simulink model "Halfcar_model_EV_simulink"  (Simulink 7.3)
settings: Solver=ode3  StartTime=0.0  StopTime=5  FixedStep=T  RelTol=1e-3
values from neighbouring files (symbols this model uses):
  v_initial = 10    [Main_for_DOCandDODR.m]
undefined symbols (not defined in the file or in its folder): a, b, cf, cr, Ds, eyeb, eyew, g, h, kf, kr, ktf, ktr, M1, M2, mb, mw, r, reduction_ratio, saturation_slipratio, step_time, T, Tdf, Tdr, wf_initial, wr_initial
libraries: simulink x2
settings Model: Creator=JSP  LastModifiedBy=JSPark

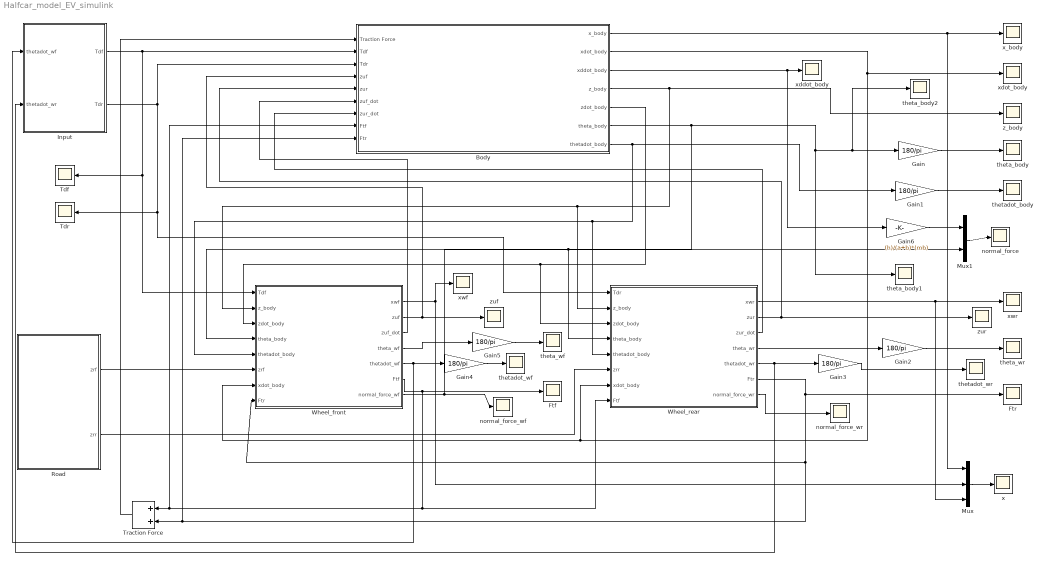
== system Halfcar_model_EV_simulink ==
  Body : Subsystem
  Ftf : Scope
      settings: YMin=1706.26  YMax=1706.26  SaveName=ScopeData11
  Ftr : Scope
      settings: SaveName=ScopeData12
  Gain{,1..5} (6 alike) : Gain  Gain=180/pi  ParameterDataType=fixdt(1, 16)  ParameterScaling=2^0  OutDataType=fixdt(1, 16)  OutScaling=2^0  SampleTime=T
  Gain6 : Gain  Gain=(h)/(a+b)*(mb)  ParameterDataType=fixdt(1, 16)  ParameterScaling=2^0  OutDataType=fixdt(1, 16)  OutScaling=2^0  SampleTime=T
  Input : Subsystem
  Mux : Mux  Inputs=3
  Mux1 : Mux  Inputs=2
  Road : Subsystem
  Tdf : Scope
      settings: YMin=-315  YMax=-285  SaveName=ScopeData24
  Tdr : Scope
      settings: SaveName=ScopeData25
  Traction Force : Sum  OutDataType=fixdt(1, 16)  OutScaling=2^-10  SampleTime=T
  Wheel_front : Subsystem
  Wheel_rear : Subsystem
  normal_force : Scope
      settings: SaveName=ScopeData33
  normal_force_wf : Scope
      settings: YMin=0  YMax=400  SaveName=ScopeData26
  normal_force_wr : Scope
      settings: SaveName=ScopeData27
  theta_body : Scope
      settings: YMin=-0.5  YMax=0  SaveName=ScopeData3
  theta_body1 : Scope
      settings: YMin=-0.5  YMax=0  SaveName=ScopeData32
  theta_body2 : Scope
      settings: YMin=-0.5  YMax=0  SaveName=ScopeData34
  theta_wf : Scope
      settings: SaveName=ScopeData8
  theta_wr : Scope
      settings: SaveName=ScopeData6
  thetadot_body : Scope
      settings: SaveName=ScopeData4
  thetadot_wf : Scope
      settings: SaveName=ScopeData18
  thetadot_wr : Scope
      settings: SaveName=ScopeData17
  x : Scope
      settings: SaveName=ScopeData13
  x_body : Scope
      settings: YMin=0  YMax=250
  xddot_body : Scope
      settings: YMin=10.125  YMax=10.45  SaveName=ScopeData28
  xdot_body : Scope
      settings: YMin=10  YMax=22
  xwf : Scope
      settings: SaveName=ScopeData9
  xwr : Scope
      settings: SaveName=ScopeData5
  z_body : Scope
      settings: YMin=0.00525  YMax=0.0075  SaveName=ScopeData2
  zuf : Scope
      settings: YMin=-1  YMax=1  SaveName=ScopeData10
  zur : Scope
      settings: SaveName=ScopeData7
  wires:
  Input/1(Tdf) -> Body/2(Tdf), Tdf/1, Wheel_front/1(Tdf)
  Input/2(Tdr) -> Body/3(Tdr), Wheel_rear/1(Tdr), Tdr/1
  Road/1(zrf) -> Wheel_front/6(zrf)
  Road/2(zrr) -> Wheel_rear/6(zrr)
  Body/4(z_body) -> Wheel_front/2(z_body), Wheel_rear/2(z_body), z_body/1
  Body/6(theta_body) -> Wheel_front/4(theta_body), Wheel_rear/4(theta_body), theta_body1/1, Gain/1, theta_body2/1
  Wheel_front/2(zuf) -> Body/4(zuf), zuf/1
  Wheel_rear/2(zur) -> Body/5(zur), zur/1
  Body/1(x_body) -> x_body/1, Mux/1
  Body/2(xdot_body) -> xdot_body/1, Wheel_front/7(xdot_body), Wheel_rear/7(xdot_body)
  Body/7(thetadot_body) -> Gain1/1, Wheel_front/5(thetadot_body), Wheel_rear/5(thetadot_body)
  Wheel_rear/1(xwr) -> xwr/1, Mux/3
  Wheel_rear/4(theta_wr) -> Gain2/1
  Wheel_front/1(xwf) -> xwf/1, Mux/2
  Wheel_front/4(theta_wf) -> Gain5/1
  Wheel_front/6(Ftf) -> Ftf/1, Wheel_rear/8(Ftf), Traction Force/1, Body/8(Ftf)
  Traction Force/1 -> Body/1(Traction Force)
  Wheel_rear/6(Ftr) -> Ftr/1, Wheel_front/8(Ftr), Traction Force/2, Body/9(Ftr)
  Mux/1 -> x/1
  Wheel_rear/5(thetadot_wr) -> Gain3/1, Input/2(thetadot_wr)
  Wheel_front/5(thetadot_wf) -> Gain4/1, Input/1(thetadot_wf)
  Gain/1 -> theta_body/1
  Gain1/1 -> thetadot_body/1
  Gain2/1 -> theta_wr/1
  Gain3/1 -> thetadot_wr/1
  Gain4/1 -> thetadot_wf/1
  Gain5/1 -> theta_wf/1
  Wheel_front/3(zuf_dot) -> Body/6(zuf_dot)
  Wheel_rear/3(zur_dot) -> Body/7(zur_dot)
  Body/5(zdot_body) -> Wheel_front/3(zdot_body), Wheel_rear/3(zdot_body)
  Wheel_front/7(normal_force_wf) -> normal_force_wf/1, Mux1/2
  Wheel_rear/7(normal_force_wr) -> normal_force_wr/1
  Body/3(xddot_body) -> xddot_body/1, Gain6/1
  Gain6/1 -> Mux1/1
  Mux1/1 -> normal_force/1

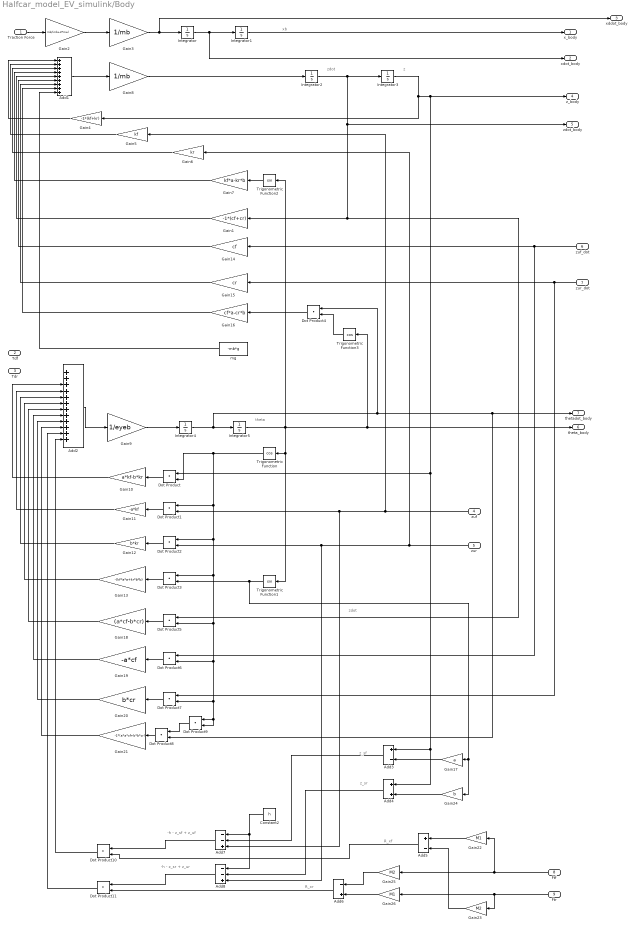
== system Halfcar_model_EV_simulink/Body ==
  note: xb
  note: z
  note: theta
  note: zdot
  note: zdot
  note: R_xf
  note: R_xr
  note: z_sf
  note: z_sr
  note: -h - z_sf + z_uf
  note: -h - z_sr + z_ur
  Traction Force : Inport
  Tdf : Inport  Port=2
  Tdr : Inport  Port=3
  zuf : Inport  Port=4
  zur : Inport  Port=5
  zuf_dot : Inport  Port=6
  zur_dot : Inport  Port=7
  Ftf : Inport  Port=8
  Ftr : Inport  Port=9
  Add1 : Sum  Inputs=+++++++++  OutDataType=fixdt(1, 16)  OutScaling=2^-10  SampleTime=T
  Add2 : Sum  Inputs=++++++++++++  OutDataType=fixdt(1, 16)  OutScaling=2^-10  SampleTime=T
  Add3 : Sum  Inputs=+-  OutDataType=fixdt(1, 16)  OutScaling=2^-10  SampleTime=T
  Add4 : Sum  OutDataType=fixdt(1, 16)  OutScaling=2^-10  SampleTime=T
  Add5 : Sum  Inputs=+-  OutDataType=fixdt(1, 16)  OutScaling=2^-10  SampleTime=T
  Add6 : Sum  Inputs=-+  OutDataType=fixdt(1, 16)  OutScaling=2^-10  SampleTime=T
  Add7 : Sum  Inputs=--+  OutDataType=fixdt(1, 16)  OutScaling=2^-10  SampleTime=T
  Add8 : Sum  Inputs=--+  OutDataType=fixdt(1, 16)  OutScaling=2^-10  SampleTime=T
  Constant2 : Constant  Value=h  OutDataType=fixdt(1, 16)  OutScaling=2^0  SampleTime=T
  Dot Product{,1..11} (12 alike) : DotProduct  SampleTime=T  OutDataType=fixdt(1, 16)  OutScaling=2^-10  InputSameDT=on  OutDataTypeStr=Inherit: Inherit via internal rule
  Gain1 : Gain  Gain=-1*(cf+cr)  ParameterDataType=fixdt(1, 16)  ParameterScaling=2^0  OutDataType=fixdt(1, 16)  OutScaling=2^0  SampleTime=T
  Gain10 : Gain  Gain=a*kf-b*kr  ParameterDataType=fixdt(1, 16)  ParameterScaling=2^0  OutDataType=fixdt(1, 16)  OutScaling=2^0  SampleTime=T
  Gain11 : Gain  Gain=-a*kf  ParameterDataType=fixdt(1, 16)  ParameterScaling=2^0  OutDataType=fixdt(1, 16)  OutScaling=2^0  SampleTime=T
  Gain12 : Gain  Gain=b*kr  ParameterDataType=fixdt(1, 16)  ParameterScaling=2^0  OutDataType=fixdt(1, 16)  OutScaling=2^0  SampleTime=T
  Gain13 : Gain  Gain=-(kf*a*a+kr*b*b)  ParameterDataType=fixdt(1, 16)  ParameterScaling=2^0  OutDataType=fixdt(1, 16)  OutScaling=2^0  SampleTime=T
  Gain14 : Gain  Gain=cf  ParameterDataType=fixdt(1, 16)  ParameterScaling=2^0  OutDataType=fixdt(1, 16)  OutScaling=2^0  SampleTime=T
  Gain15 : Gain  Gain=cr  ParameterDataType=fixdt(1, 16)  ParameterScaling=2^0  OutDataType=fixdt(1, 16)  OutScaling=2^0  SampleTime=T
  Gain16 : Gain  Gain=cf*a-cr*b  ParameterDataType=fixdt(1, 16)  ParameterScaling=2^0  OutDataType=fixdt(1, 16)  OutScaling=2^0  SampleTime=T
  Gain17 : Gain  Gain=a  ParameterDataType=fixdt(1, 16)  ParameterScaling=2^0  OutDataType=fixdt(1, 16)  OutScaling=2^0  SampleTime=T
  Gain18 : Gain  Gain=(a*cf-b*cr)  ParameterDataType=fixdt(1, 16)  ParameterScaling=2^0  OutDataType=fixdt(1, 16)  OutScaling=2^0  SampleTime=T
  Gain19 : Gain  Gain=-a*cf  ParameterDataType=fixdt(1, 16)  ParameterScaling=2^0  OutDataType=fixdt(1, 16)  OutScaling=2^0  SampleTime=T
  Gain2 : Gain  Gain=mb/(mb+2*mw)  ParameterDataType=fixdt(1, 16)  ParameterScaling=2^0  OutDataType=fixdt(1, 16)  OutScaling=2^0  SampleTime=T
  Gain20 : Gain  Gain=b*cr  ParameterDataType=fixdt(1, 16)  ParameterScaling=2^0  OutDataType=fixdt(1, 16)  OutScaling=2^0  SampleTime=T
  Gain21 : Gain  Gain=-1*(a*a*cf+b*b*cr)  ParameterDataType=fixdt(1, 16)  ParameterScaling=2^0  OutDataType=fixdt(1, 16)  OutScaling=2^0  SampleTime=T
  Gain22 : Gain  Gain=M1  ParameterDataType=fixdt(1, 16)  ParameterScaling=2^0  OutDataType=fixdt(1, 16)  OutScaling=2^0  SampleTime=T
  Gain23 : Gain  Gain=M2  ParameterDataType=fixdt(1, 16)  ParameterScaling=2^0  OutDataType=fixdt(1, 16)  OutScaling=2^0  SampleTime=T
  Gain24 : Gain  Gain=b  ParameterDataType=fixdt(1, 16)  ParameterScaling=2^0  OutDataType=fixdt(1, 16)  OutScaling=2^0  SampleTime=T
  Gain25 : Gain  Gain=M2  ParameterDataType=fixdt(1, 16)  ParameterScaling=2^0  OutDataType=fixdt(1, 16)  OutScaling=2^0  SampleTime=T
  Gain26 : Gain  Gain=M1  ParameterDataType=fixdt(1, 16)  ParameterScaling=2^0  OutDataType=fixdt(1, 16)  OutScaling=2^0  SampleTime=T
  Gain3 : Gain  Gain=1/mb  ParameterDataType=fixdt(1, 16)  ParameterScaling=2^0  OutDataType=fixdt(1, 16)  OutScaling=2^0  SampleTime=T
  Gain4 : Gain  Gain=-1*(kf+kr)  ParameterDataType=fixdt(1, 16)  ParameterScaling=2^0  OutDataType=fixdt(1, 16)  OutScaling=2^0  SampleTime=T
  Gain5 : Gain  Gain=kf  ParameterDataType=fixdt(1, 16)  ParameterScaling=2^0  OutDataType=fixdt(1, 16)  OutScaling=2^0  SampleTime=T
  Gain6 : Gain  Gain=kr  ParameterDataType=fixdt(1, 16)  ParameterScaling=2^0  OutDataType=fixdt(1, 16)  OutScaling=2^0  SampleTime=T
  Gain7 : Gain  Gain=kf*a-kr*b  ParameterDataType=fixdt(1, 16)  ParameterScaling=2^0  OutDataType=fixdt(1, 16)  OutScaling=2^0  SampleTime=T
  Gain8 : Gain  Gain=1/mb  ParameterDataType=fixdt(1, 16)  ParameterScaling=2^0  OutDataType=fixdt(1, 16)  OutScaling=2^0  SampleTime=T
  Gain9 : Gain  Gain=1/eyeb  ParameterDataType=fixdt(1, 16)  ParameterScaling=2^0  OutDataType=fixdt(1, 16)  OutScaling=2^0  SampleTime=T
  Integrator : Integrator  InitialCondition=v_initial
  Integrator{1..5} (5 alike) : Integrator
  Trigonometric Function : Trigonometry  Operator=cos  SampleTime=T
  Trigonometric Function1 : Trigonometry  SampleTime=T
  Trigonometric Function2 : Trigonometry  SampleTime=T
  Trigonometric Function3 : Trigonometry  Operator=cos  SampleTime=T
  mg : Constant  Value=-mb*g  OutDataType=fixdt(1, 16)  OutScaling=2^0  SampleTime=T
  x_body : Outport
  xdot_body : Outport  Port=2
  xddot_body : Outport  Port=3
  z_body : Outport  Port=4
  zdot_body : Outport  Port=5
  theta_body : Outport  Port=6
  thetadot_body : Outport  Port=7
  wires:
  Gain2/1 -> Gain3/1
  Gain3/1 -> Integrator/1, xddot_body/1
  Integrator/1 -> Integrator1/1, xdot_body/1
  Gain8/1 -> Integrator2/1
  Integrator2/1 -> Integrator3/1, Gain1/1, Dot Product5/1, zdot_body/1
  Add1/1 -> Gain8/1
  Gain4/1 -> Add1/1
  Gain5/1 -> Add1/2
  Gain6/1 -> Add1/3
  Gain7/1 -> Add1/4
  Integrator3/1 -> Gain4/1, z_body/1, Dot Product/1, Add3/1, Add4/1
  Gain9/1 -> Integrator4/1
  Integrator4/1 -> Integrator5/1, Dot Product4/1, thetadot_body/1, Dot Product8/2
  Dot Product/1 -> Gain10/1
  Integrator5/1 -> Trigonometric Function/1, Trigonometric Function1/1, Trigonometric Function2/1, theta_body/1, Trigonometric Function3/1
  Trigonometric Function/1 -> Dot Product/2, Dot Product1/1, Dot Product2/1, Dot Product3/1, Dot Product5/2, Dot Product6/2, Dot Product7/2, Dot Product9/1, Dot Product9/2
  Add2/1 -> Gain9/1
  Gain10/1 -> Add2/3
  Dot Product1/1 -> Gain11/1
  Dot Product2/1 -> Gain12/1
  Trigonometric Function1/1 -> Dot Product3/2, Gain17/1, Gain24/1
  Dot Product3/1 -> Gain13/1
  Gain13/1 -> Add2/6
  Gain11/1 -> Add2/4
  Gain12/1 -> Add2/5
  Integrator1/1 -> x_body/1
  Trigonometric Function2/1 -> Gain7/1
  zur/1 -> Gain6/1, Dot Product2/2, Add8/3
  Traction Force/1 -> Gain2/1
  zuf/1 -> Gain5/1, Dot Product1/2, Add7/3
  zuf_dot/1 -> Gain14/1, Dot Product6/1
  zur_dot/1 -> Gain15/1, Dot Product7/1
  Dot Product4/1 -> Gain16/1
  Trigonometric Function3/1 -> Dot Product4/2
  Gain1/1 -> Add1/5
  Gain14/1 -> Add1/6
  Gain15/1 -> Add1/7
  Gain16/1 -> Add1/8
  mg/1 -> Add1/9
  Dot Product5/1 -> Gain18/1
  Dot Product6/1 -> Gain19/1
  Dot Product7/1 -> Gain20/1
  Dot Product9/1 -> Dot Product8/1
  Dot Product8/1 -> Gain21/1
  Gain18/1 -> Add2/7
  Gain19/1 -> Add2/8
  Gain20/1 -> Add2/9
  Gain21/1 -> Add2/10
  Ftf/1 -> Gain22/1, Gain25/1
  Ftr/1 -> Gain23/1, Gain26/1
  Gain22/1 -> Add5/1
  Gain23/1 -> Add5/2
  Gain25/1 -> Add6/1
  Gain26/1 -> Add6/2
  Constant2/1 -> Add7/1, Add8/1
  Add7/1 -> Dot Product10/1
  Add5/1 -> Dot Product10/2
  Add8/1 -> Dot Product11/1
  Add6/1 -> Dot Product11/2
  Gain24/1 -> Add4/2
  Gain17/1 -> Add3/2
  Add3/1 -> Add7/2
  Add4/1 -> Add8/2
  Dot Product10/1 -> Add2/12
  Dot Product11/1 -> Add2/11

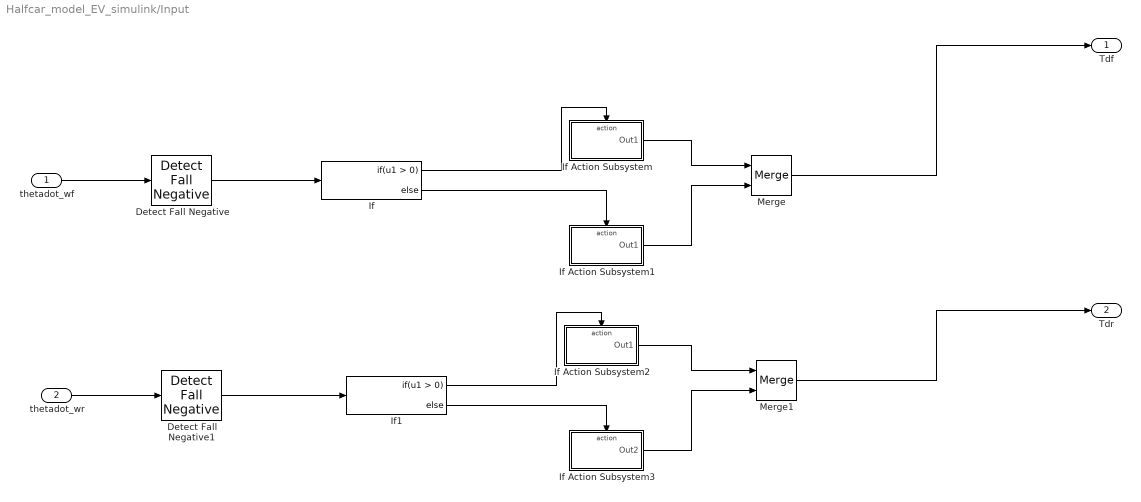
== system Halfcar_model_EV_simulink/Input ==
  thetadot_wf : Inport
  thetadot_wr : Inport  Port=2
  Detect Fall Negative : simulink/Logic and Bit Operations/Detect Fall Negative  SystemSampleTime=-1  vinit=0
  Detect Fall Negative1 : simulink/Logic and Bit Operations/Detect Fall Negative  SystemSampleTime=-1  vinit=0
  If : If  SampleTime=T
  If Action Subsystem : Subsystem  TreatAsAtomicUnit=on
  If Action Subsystem1 : Subsystem  TreatAsAtomicUnit=on
  If Action Subsystem2 : Subsystem  TreatAsAtomicUnit=on
  If Action Subsystem3 : Subsystem  TreatAsAtomicUnit=on
  If1 : If  SampleTime=T
  Merge : Merge  InitialOutput=0
  Merge1 : Merge  InitialOutput=0
  Tdf : Outport
  Tdr : Outport  Port=2
  wires:
  thetadot_wf/1 -> Detect Fall Negative/1
  If/1 -> If Action Subsystem/Action
  If/2 -> If Action Subsystem1/Action
  If Action Subsystem/1(Out1) -> Merge/1
  If Action Subsystem1/1(Out1) -> Merge/2
  Merge/1 -> Tdf/1
  If1/1 -> If Action Subsystem2/Action
  If1/2 -> If Action Subsystem3/Action
  If Action Subsystem2/1(Out1) -> Merge1/1
  If Action Subsystem3/1(Out2) -> Merge1/2
  Merge1/1 -> Tdr/1
  thetadot_wr/1 -> Detect Fall Negative1/1
  Detect Fall Negative/1 -> If/1
  Detect Fall Negative1/1 -> If1/1

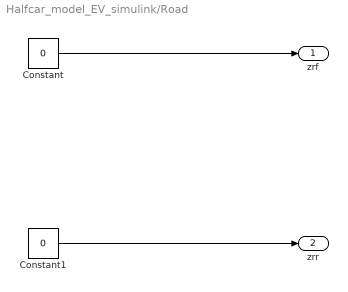
== system Halfcar_model_EV_simulink/Road ==
  Constant : Constant  Value=0  OutDataType=fixdt(1, 16)  OutScaling=2^0  SampleTime=T
  Constant1 : Constant  Value=0  OutDataType=fixdt(1, 16)  OutScaling=2^0  SampleTime=T
  zrf : Outport
  zrr : Outport  Port=2
  wires:
  Constant/1 -> zrf/1
  Constant1/1 -> zrr/1

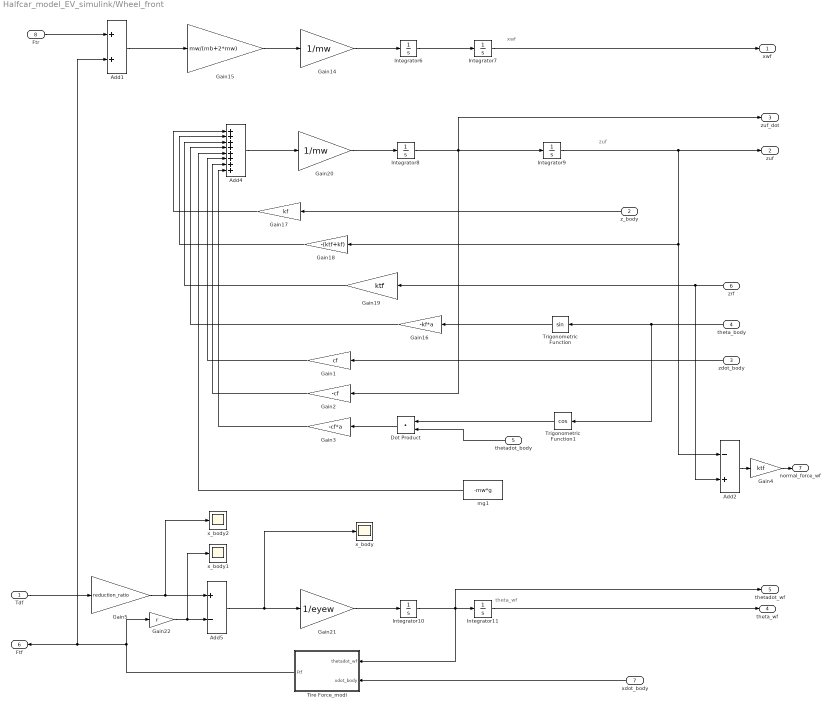
== system Halfcar_model_EV_simulink/Wheel_front ==
  note: xwf
  note: zuf
  note: theta_wf
  Tdf : Inport
  z_body : Inport  Port=2
  zdot_body : Inport  Port=3
  theta_body : Inport  Port=4
  thetadot_body : Inport  Port=5
  zrf : Inport  Port=6
  xdot_body : Inport  Port=7
  Ftr : Inport  Port=8
  Add1 : Sum  OutDataType=fixdt(1, 16)  OutScaling=2^-10  SampleTime=T
  Add2 : Sum  Inputs=-+  OutDataType=fixdt(1, 16)  OutScaling=2^-10  SampleTime=T
  Add4 : Sum  Inputs=++++++++  OutDataType=fixdt(1, 16)  OutScaling=2^-10  SampleTime=T
  Add5 : Sum  Inputs=+-  OutDataType=fixdt(1, 16)  OutScaling=2^-10  SampleTime=T
  Dot Product : DotProduct  SampleTime=T  OutDataType=fixdt(1, 16)  OutScaling=2^-10  InputSameDT=on  OutDataTypeStr=Inherit: Inherit via internal rule
  Gain1 : Gain  Gain=cf  ParameterDataType=fixdt(1, 16)  ParameterScaling=2^0  OutDataType=fixdt(1, 16)  OutScaling=2^0  SampleTime=T
  Gain14 : Gain  Gain=1/mw  ParameterDataType=fixdt(1, 16)  ParameterScaling=2^0  OutDataType=fixdt(1, 16)  OutScaling=2^0  SampleTime=T
  Gain15 : Gain  Gain=mw/(mb+2*mw)  ParameterDataType=fixdt(1, 16)  ParameterScaling=2^0  OutDataType=fixdt(1, 16)  OutScaling=2^0  SampleTime=T
  Gain16 : Gain  Gain=-kf*a  ParameterDataType=fixdt(1, 16)  ParameterScaling=2^0  OutDataType=fixdt(1, 16)  OutScaling=2^0  SampleTime=T
  Gain17 : Gain  Gain=kf  ParameterDataType=fixdt(1, 16)  ParameterScaling=2^0  OutDataType=fixdt(1, 16)  OutScaling=2^0  SampleTime=T
  Gain18 : Gain  Gain=-(ktf+kf)  ParameterDataType=fixdt(1, 16)  ParameterScaling=2^0  OutDataType=fixdt(1, 16)  OutScaling=2^0  SampleTime=T
  Gain19 : Gain  Gain=ktf  ParameterDataType=fixdt(1, 16)  ParameterScaling=2^0  OutDataType=fixdt(1, 16)  OutScaling=2^0  SampleTime=T
  Gain2 : Gain  Gain=-cf  ParameterDataType=fixdt(1, 16)  ParameterScaling=2^0  OutDataType=fixdt(1, 16)  OutScaling=2^0  SampleTime=T
  Gain20 : Gain  Gain=1/mw  ParameterDataType=fixdt(1, 16)  ParameterScaling=2^0  OutDataType=fixdt(1, 16)  OutScaling=2^0  SampleTime=T
  Gain21 : Gain  Gain=1/eyew  ParameterDataType=fixdt(1, 16)  ParameterScaling=2^0  OutDataType=fixdt(1, 16)  OutScaling=2^0  SampleTime=T
  Gain22 : Gain  Gain=r  ParameterDataType=fixdt(1, 16)  ParameterScaling=2^0  OutDataType=fixdt(1, 16)  OutScaling=2^0  SampleTime=T
  Gain3 : Gain  Gain=-cf*a  ParameterDataType=fixdt(1, 16)  ParameterScaling=2^0  OutDataType=fixdt(1, 16)  OutScaling=2^0  SampleTime=T
  Gain4 : Gain  Gain=ktf  ParameterDataType=fixdt(1, 16)  ParameterScaling=2^0  OutDataType=fixdt(1, 16)  OutScaling=2^0  SampleTime=T
  Gain5 : Gain  Gain=reduction_ratio  ParameterDataType=fixdt(1, 16)  ParameterScaling=2^0  OutDataType=fixdt(1, 16)  OutScaling=2^0  SampleTime=T
  Integrator10 : Integrator  InitialCondition=wf_initial
  Integrator{7..9,11} (4 alike) : Integrator
  Integrator6 : Integrator  InitialCondition=v_initial
  Tire Force_modi : Subsystem
  Trigonometric Function : Trigonometry  SampleTime=T
  Trigonometric Function1 : Trigonometry  Operator=cos  SampleTime=T
  mg1 : Constant  Value=-mw*g  OutDataType=fixdt(1, 16)  OutScaling=2^0  SampleTime=T
  x_body : Scope
      settings: YMin=0  YMax=100  SaveName=ScopeData16
  x_body1 : Scope
      settings: SaveName=ScopeData30
  x_body2 : Scope
      settings: SaveName=ScopeData31
  xwf : Outport
  zuf : Outport  Port=2
  zuf_dot : Outport  Port=3
  theta_wf : Outport  Port=4
  thetadot_wf : Outport  Port=5
  Ftf : Outport  Port=6
  normal_force_wf : Outport  Port=7
  wires:
  Gain15/1 -> Gain14/1
  Gain14/1 -> Integrator6/1
  Integrator6/1 -> Integrator7/1
  Gain20/1 -> Integrator8/1
  Integrator8/1 -> Integrator9/1, zuf_dot/1, Gain2/1
  Add4/1 -> Gain20/1
  Gain17/1 -> Add4/1
  Gain18/1 -> Add4/2
  Gain19/1 -> Add4/3
  Gain16/1 -> Add4/4
  mg1/1 -> Add4/5
  Gain21/1 -> Integrator10/1
  Integrator10/1 -> Integrator11/1, thetadot_wf/1, Tire Force_modi/1(thetadot_wf)
  Add5/1 -> Gain21/1, x_body/1
  Gain22/1 -> Add5/2, x_body1/1
  Integrator7/1 -> xwf/1
  Integrator9/1 -> zuf/1, Gain18/1, Add2/1
  Integrator11/1 -> theta_wf/1
  zrf/1 -> Gain19/1, Add2/2
  z_body/1 -> Gain17/1
  theta_body/1 -> Trigonometric Function/1, Trigonometric Function1/1
  Trigonometric Function/1 -> Gain16/1
  xdot_body/1 -> Tire Force_modi/2(xdot_body)
  Tdf/1 -> Gain5/1
  Tire Force_modi/1(Ftf) -> Ftf/1, Add1/2, Gain22/1
  Ftr/1 -> Add1/1
  Add1/1 -> Gain15/1
  zdot_body/1 -> Gain1/1
  Dot Product/1 -> Gain3/1
  Trigonometric Function1/1 -> Dot Product/1
  thetadot_body/1 -> Dot Product/2
  Gain1/1 -> Add4/6
  Gain2/1 -> Add4/7
  Gain3/1 -> Add4/8
  Add2/1 -> Gain4/1
  Gain4/1 -> normal_force_wf/1
  Gain5/1 -> Add5/1, x_body2/1

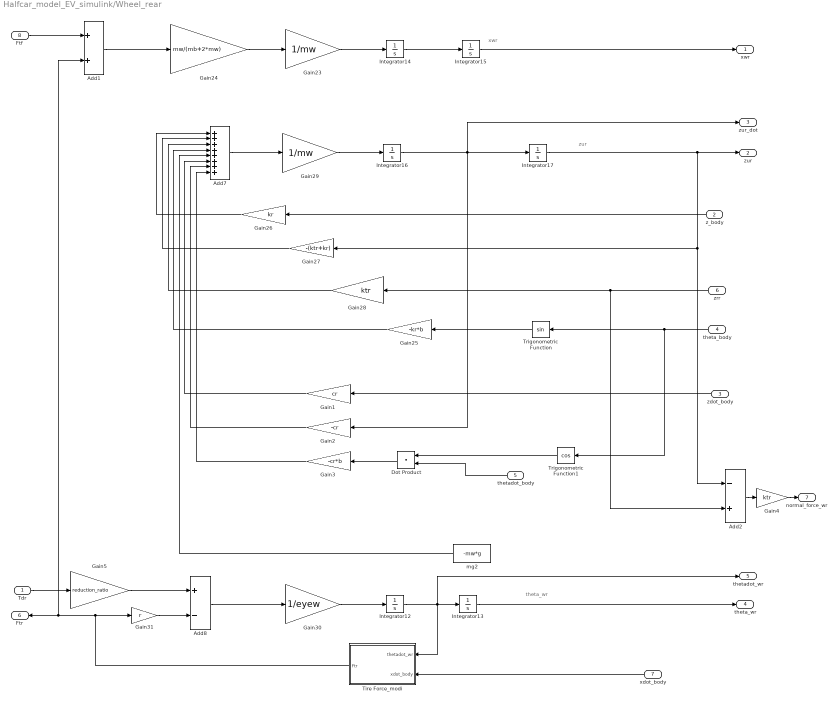
== system Halfcar_model_EV_simulink/Wheel_rear ==
  note: xwr
  note: zur
  note: theta_wr
  Tdr : Inport
  z_body : Inport  Port=2
  zdot_body : Inport  Port=3
  theta_body : Inport  Port=4
  thetadot_body : Inport  Port=5
  zrr : Inport  Port=6
  xdot_body : Inport  Port=7
  Ftf : Inport  Port=8
  Add1 : Sum  OutDataType=fixdt(1, 16)  OutScaling=2^-10  SampleTime=T
  Add2 : Sum  Inputs=-+  OutDataType=fixdt(1, 16)  OutScaling=2^-10  SampleTime=T
  Add7 : Sum  Inputs=++++++++  OutDataType=fixdt(1, 16)  OutScaling=2^-10  SampleTime=T
  Add8 : Sum  Inputs=+-  OutDataType=fixdt(1, 16)  OutScaling=2^-10  SampleTime=T
  Dot Product : DotProduct  SampleTime=T  OutDataType=fixdt(1, 16)  OutScaling=2^-10  InputSameDT=on  OutDataTypeStr=Inherit: Inherit via internal rule
  Gain1 : Gain  Gain=cr  ParameterDataType=fixdt(1, 16)  ParameterScaling=2^0  OutDataType=fixdt(1, 16)  OutScaling=2^0  SampleTime=T
  Gain2 : Gain  Gain=-cr  ParameterDataType=fixdt(1, 16)  ParameterScaling=2^0  OutDataType=fixdt(1, 16)  OutScaling=2^0  SampleTime=T
  Gain23 : Gain  Gain=1/mw  ParameterDataType=fixdt(1, 16)  ParameterScaling=2^0  OutDataType=fixdt(1, 16)  OutScaling=2^0  SampleTime=T
  Gain24 : Gain  Gain=mw/(mb+2*mw)  ParameterDataType=fixdt(1, 16)  ParameterScaling=2^0  OutDataType=fixdt(1, 16)  OutScaling=2^0  SampleTime=T
  Gain25 : Gain  Gain=-kr*b  ParameterDataType=fixdt(1, 16)  ParameterScaling=2^0  OutDataType=fixdt(1, 16)  OutScaling=2^0  SampleTime=T
  Gain26 : Gain  Gain=kr  ParameterDataType=fixdt(1, 16)  ParameterScaling=2^0  OutDataType=fixdt(1, 16)  OutScaling=2^0  SampleTime=T
  Gain27 : Gain  Gain=-(ktr+kr)  ParameterDataType=fixdt(1, 16)  ParameterScaling=2^0  OutDataType=fixdt(1, 16)  OutScaling=2^0  SampleTime=T
  Gain28 : Gain  Gain=ktr  ParameterDataType=fixdt(1, 16)  ParameterScaling=2^0  OutDataType=fixdt(1, 16)  OutScaling=2^0  SampleTime=T
  Gain29 : Gain  Gain=1/mw  ParameterDataType=fixdt(1, 16)  ParameterScaling=2^0  OutDataType=fixdt(1, 16)  OutScaling=2^0  SampleTime=T
  Gain3 : Gain  Gain=-cr*b  ParameterDataType=fixdt(1, 16)  ParameterScaling=2^0  OutDataType=fixdt(1, 16)  OutScaling=2^0  SampleTime=T
  Gain30 : Gain  Gain=1/eyew  ParameterDataType=fixdt(1, 16)  ParameterScaling=2^0  OutDataType=fixdt(1, 16)  OutScaling=2^0  SampleTime=T
  Gain31 : Gain  Gain=r  ParameterDataType=fixdt(1, 16)  ParameterScaling=2^0  OutDataType=fixdt(1, 16)  OutScaling=2^0  SampleTime=T
  Gain4 : Gain  Gain=ktr  ParameterDataType=fixdt(1, 16)  ParameterScaling=2^0  OutDataType=fixdt(1, 16)  OutScaling=2^0  SampleTime=T
  Gain5 : Gain  Gain=reduction_ratio  ParameterDataType=fixdt(1, 16)  ParameterScaling=2^0  OutDataType=fixdt(1, 16)  OutScaling=2^0  SampleTime=T
  Integrator12 : Integrator  InitialCondition=wr_initial
  Integrator{13,15..17} (4 alike) : Integrator
  Integrator14 : Integrator  InitialCondition=v_initial
  Tire Force_modi : Subsystem
  Trigonometric Function : Trigonometry  SampleTime=T
  Trigonometric Function1 : Trigonometry  Operator=cos  SampleTime=T
  mg2 : Constant  Value=-mw*g  OutDataType=fixdt(1, 16)  OutScaling=2^0  SampleTime=T
  xwr : Outport
  zur : Outport  Port=2
  zur_dot : Outport  Port=3
  theta_wr : Outport  Port=4
  thetadot_wr : Outport  Port=5
  Ftr : Outport  Port=6
  normal_force_wr : Outport  Port=7
  wires:
  Gain24/1 -> Gain23/1
  Gain23/1 -> Integrator14/1
  Integrator14/1 -> Integrator15/1
  Gain29/1 -> Integrator16/1
  Integrator16/1 -> Integrator17/1, zur_dot/1, Gain2/1
  Add7/1 -> Gain29/1
  Gain26/1 -> Add7/1
  Gain27/1 -> Add7/2
  Gain28/1 -> Add7/3
  Gain25/1 -> Add7/4
  mg2/1 -> Add7/5
  Gain30/1 -> Integrator12/1
  Integrator12/1 -> Integrator13/1, thetadot_wr/1, Tire Force_modi/1(thetadot_wr)
  Add8/1 -> Gain30/1
  Gain31/1 -> Add8/2
  Integrator15/1 -> xwr/1
  Integrator17/1 -> zur/1, Gain27/1, Add2/1
  Integrator13/1 -> theta_wr/1
  zrr/1 -> Gain28/1, Add2/2
  z_body/1 -> Gain26/1
  theta_body/1 -> Trigonometric Function/1, Trigonometric Function1/1
  Tdr/1 -> Gain5/1
  Trigonometric Function/1 -> Gain25/1
  Tire Force_modi/1(Ftr) -> Ftr/1, Add1/2, Gain31/1
  Add1/1 -> Gain24/1
  Ftf/1 -> Add1/1
  xdot_body/1 -> Tire Force_modi/2(xdot_body)
  zdot_body/1 -> Gain1/1
  Dot Product/1 -> Gain3/1
  Trigonometric Function1/1 -> Dot Product/1
  thetadot_body/1 -> Dot Product/2
  Gain1/1 -> Add7/6
  Gain2/1 -> Add7/7
  Gain3/1 -> Add7/8
  Add2/1 -> Gain4/1
  Gain4/1 -> normal_force_wr/1
  Gain5/1 -> Add8/1

== system Halfcar_model_EV_simulink/Input/If Action Subsystem ==
  Action Port : ActionPort  ActionType=then
  Constant : Constant  Value=0  OutDataType=fixdt(1, 16)  OutScaling=2^0  SampleTime=T
  Out1 : Outport  OutDataType=fixdt(1, 16)  OutScaling=2^0  InitialOutput=0
  wires:
  Constant/1 -> Out1/1

== system Halfcar_model_EV_simulink/Input/If Action Subsystem1 ==
  Action Port : ActionPort  ActionType=else
  Tdf_1 : Step  Time=step_time  After=Tdf  SampleTime=T
  Out1 : Outport  OutDataType=fixdt(1, 16)  OutScaling=2^0  InitialOutput=0
  wires:
  Tdf_1/1 -> Out1/1

== system Halfcar_model_EV_simulink/Input/If Action Subsystem2 ==
  Action Port : ActionPort  ActionType=then
  Constant : Constant  Value=0  OutDataType=fixdt(1, 16)  OutScaling=2^0  SampleTime=T
  Out1 : Outport  OutDataType=fixdt(1, 16)  OutScaling=2^0  InitialOutput=0
  wires:
  Constant/1 -> Out1/1

== system Halfcar_model_EV_simulink/Input/If Action Subsystem3 ==
  Action Port : ActionPort  ActionType=else
  Tdr_2 : Step  Time=step_time  After=Tdr  SampleTime=T
  Out2 : Outport  OutDataType=fixdt(1, 16)  OutScaling=2^0  InitialOutput=0
  wires:
  Tdr_2/1 -> Out2/1

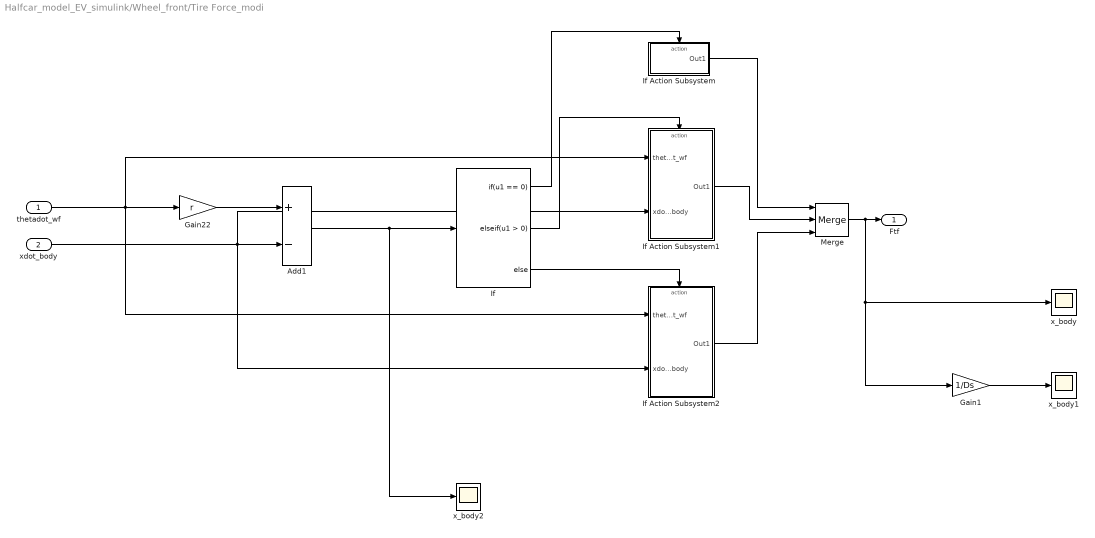
== system Halfcar_model_EV_simulink/Wheel_front/Tire Force_modi ==
  thetadot_wf : Inport
  xdot_body : Inport  Port=2
  Add1 : Sum  Inputs=+-  OutDataType=fixdt(1, 16)  OutScaling=2^-10  SampleTime=T
  Gain1 : Gain  Gain=1/Ds  ParameterDataType=fixdt(1, 16)  ParameterScaling=2^0  OutDataType=fixdt(1, 16)  OutScaling=2^0  SampleTime=T
  Gain22 : Gain  Gain=r  ParameterDataType=fixdt(1, 16)  ParameterScaling=2^0  OutDataType=fixdt(1, 16)  OutScaling=2^0  SampleTime=T
  If : If  IfExpression=u1 == 0  ElseIfExpressions=u1 > 0  SampleTime=T
  If Action Subsystem : Subsystem  TreatAsAtomicUnit=on
  If Action Subsystem1 : Subsystem  TreatAsAtomicUnit=on
  If Action Subsystem2 : Subsystem  TreatAsAtomicUnit=on
  Merge : Merge  Inputs=3  InitialOutput=0
  x_body : Scope
      settings: SaveName=ScopeData19
  x_body1 : Scope
      settings: SaveName=ScopeData14
  x_body2 : Scope
      settings: SaveName=ScopeData15
  Ftf : Outport
  wires:
  xdot_body/1 -> Add1/2, If Action Subsystem1/2(xdot_body), If Action Subsystem2/2(xdot_body)
  thetadot_wf/1 -> Gain22/1, If Action Subsystem1/1(thetadot_wf), If Action Subsystem2/1(thetadot_wf)
  Gain22/1 -> Add1/1
  Add1/1 -> If/1, x_body2/1
  If Action Subsystem/1(Out1) -> Merge/1
  If/1 -> If Action Subsystem/Action
  If/2 -> If Action Subsystem1/Action
  If/3 -> If Action Subsystem2/Action
  If Action Subsystem1/1(Out1) -> Merge/2
  If Action Subsystem2/1(Out1) -> Merge/3
  Merge/1 -> Ftf/1, x_body/1, Gain1/1
  Gain1/1 -> x_body1/1

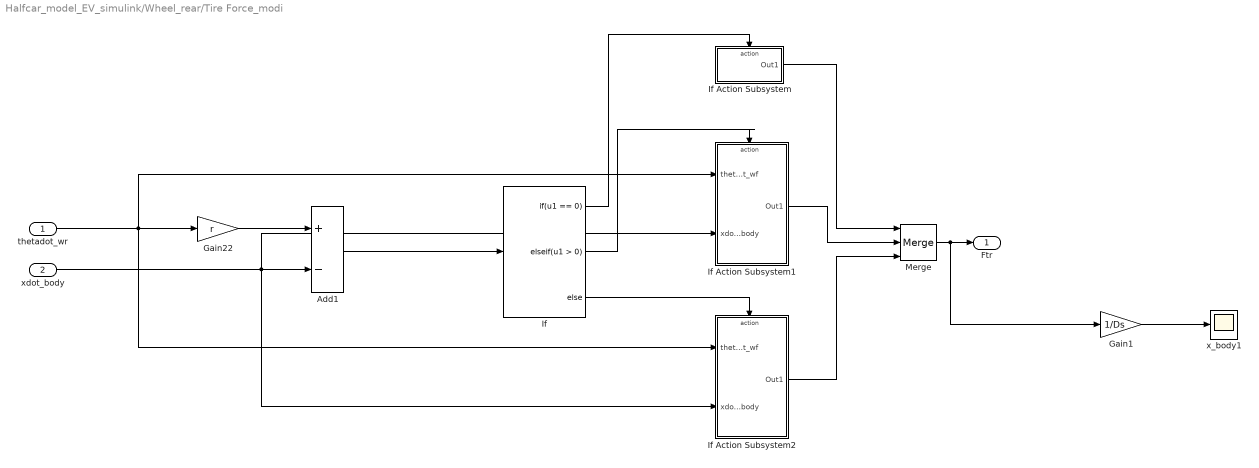
== system Halfcar_model_EV_simulink/Wheel_rear/Tire Force_modi ==
  thetadot_wr : Inport
  xdot_body : Inport  Port=2
  Add1 : Sum  Inputs=+-  OutDataType=fixdt(1, 16)  OutScaling=2^-10  SampleTime=T
  Gain1 : Gain  Gain=1/Ds  ParameterDataType=fixdt(1, 16)  ParameterScaling=2^0  OutDataType=fixdt(1, 16)  OutScaling=2^0  SampleTime=T
  Gain22 : Gain  Gain=r  ParameterDataType=fixdt(1, 16)  ParameterScaling=2^0  OutDataType=fixdt(1, 16)  OutScaling=2^0  SampleTime=T
  If : If  IfExpression=u1 == 0  ElseIfExpressions=u1 > 0  SampleTime=T
  If Action Subsystem : Subsystem  TreatAsAtomicUnit=on
  If Action Subsystem1 : Subsystem  TreatAsAtomicUnit=on
  If Action Subsystem2 : Subsystem  TreatAsAtomicUnit=on
  Merge : Merge  Inputs=3  InitialOutput=0
  x_body1 : Scope
      settings: SaveName=ScopeData37
  Ftr : Outport
  wires:
  xdot_body/1 -> Add1/2, If Action Subsystem1/2(xdot_body), If Action Subsystem2/2(xdot_body)
  thetadot_wr/1 -> Gain22/1, If Action Subsystem1/1(thetadot_wf), If Action Subsystem2/1(thetadot_wf)
  Gain22/1 -> Add1/1
  Add1/1 -> If/1
  If Action Subsystem/1(Out1) -> Merge/1
  If/1 -> If Action Subsystem/Action
  If/2 -> If Action Subsystem1/Action
  If/3 -> If Action Subsystem2/Action
  If Action Subsystem1/1(Out1) -> Merge/2
  If Action Subsystem2/1(Out1) -> Merge/3
  Merge/1 -> Ftr/1, Gain1/1
  Gain1/1 -> x_body1/1

== system Halfcar_model_EV_simulink/Wheel_front/Tire Force_modi/If Action Subsystem ==
  Action Port : ActionPort  ActionType=then
  Constant : Constant  Value=0  OutDataType=fixdt(1, 16)  OutScaling=2^0  SampleTime=T
  Out1 : Outport  OutDataType=fixdt(1, 16)  OutScaling=2^0  InitialOutput=0
  wires:
  Constant/1 -> Out1/1

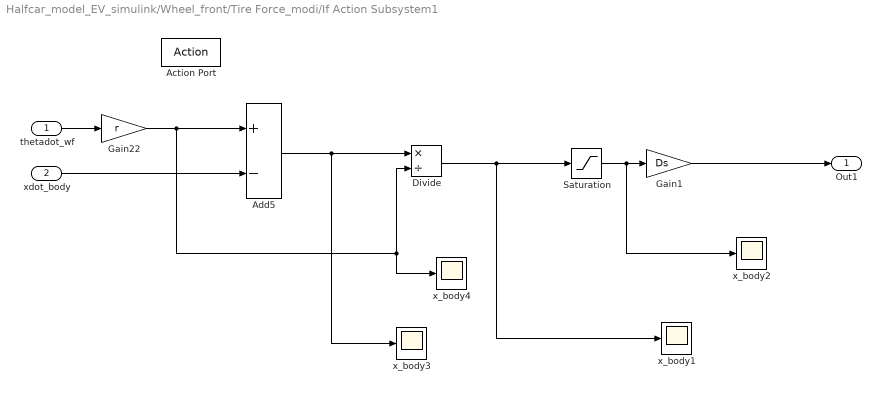
== system Halfcar_model_EV_simulink/Wheel_front/Tire Force_modi/If Action Subsystem1 ==
  thetadot_wf : Inport
  xdot_body : Inport  Port=2
  Action Port : ActionPort  ActionType=elseif
  Add5 : Sum  Inputs=+-  OutDataType=fixdt(1, 16)  OutScaling=2^-10  SampleTime=T
  Divide : Product  Inputs=*/  OutDataType=fixdt(1, 16)  OutScaling=2^-10  SampleTime=T
  Gain1 : Gain  Gain=Ds  ParameterDataType=fixdt(1, 16)  ParameterScaling=2^0  OutDataType=fixdt(1, 16)  OutScaling=2^0  SampleTime=T
  Gain22 : Gain  Gain=r  ParameterDataType=fixdt(1, 16)  ParameterScaling=2^0  OutDataType=fixdt(1, 16)  OutScaling=2^0  SampleTime=T
  Saturation : Saturate  UpperLimit=saturation_slipratio  LowerLimit=-saturation_slipratio  SampleTime=T  OutDataType=fixdt(1, 16)  OutScaling=2^0
  x_body{1..4} (4 alike) : Scope
      x_body1 settings: SaveName=ScopeData20
      x_body2 settings: SaveName=ScopeData21
      x_body3 settings: SaveName=ScopeData22
      x_body4 settings: SaveName=ScopeData23
  Out1 : Outport  OutDataType=fixdt(1, 16)  OutScaling=2^0  InitialOutput=0
  wires:
  thetadot_wf/1 -> Gain22/1
  xdot_body/1 -> Add5/2
  Add5/1 -> Divide/1, x_body3/1
  Divide/1 -> Saturation/1, x_body1/1
  Gain22/1 -> Add5/1, Divide/2, x_body4/1
  Saturation/1 -> Gain1/1, x_body2/1
  Gain1/1 -> Out1/1

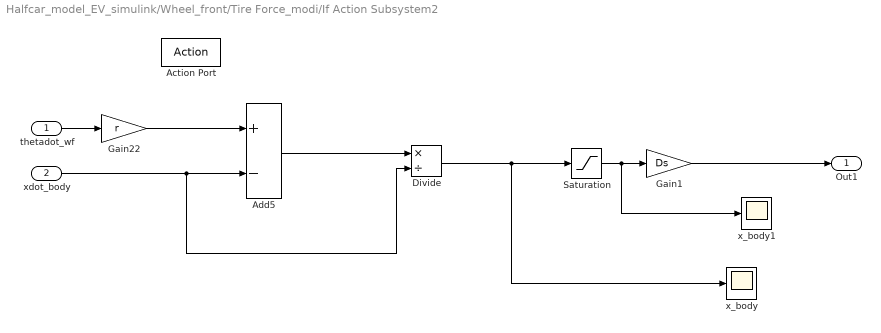
== system Halfcar_model_EV_simulink/Wheel_front/Tire Force_modi/If Action Subsystem2 ==
  thetadot_wf : Inport
  xdot_body : Inport  Port=2
  Action Port : ActionPort  ActionType=else
  Add5 : Sum  Inputs=+-  OutDataType=fixdt(1, 16)  OutScaling=2^-10  SampleTime=T
  Divide : Product  Inputs=*/  OutDataType=fixdt(1, 16)  OutScaling=2^-10  SampleTime=T
  Gain1 : Gain  Gain=Ds  ParameterDataType=fixdt(1, 16)  ParameterScaling=2^0  OutDataType=fixdt(1, 16)  OutScaling=2^0  SampleTime=T
  Gain22 : Gain  Gain=r  ParameterDataType=fixdt(1, 16)  ParameterScaling=2^0  OutDataType=fixdt(1, 16)  OutScaling=2^0  SampleTime=T
  Saturation : Saturate  UpperLimit=saturation_slipratio  LowerLimit=-saturation_slipratio  SampleTime=T  OutDataType=fixdt(1, 16)  OutScaling=2^0
  x_body : Scope
      settings: SaveName=ScopeData29
  x_body1 : Scope
      settings: SaveName=ScopeData36
  Out1 : Outport  OutDataType=fixdt(1, 16)  OutScaling=2^0  InitialOutput=0
  wires:
  Gain1/1 -> Out1/1
  Saturation/1 -> Gain1/1, x_body1/1
  Gain22/1 -> Add5/1
  Divide/1 -> Saturation/1, x_body/1
  Add5/1 -> Divide/1
  xdot_body/1 -> Add5/2, Divide/2
  thetadot_wf/1 -> Gain22/1

== system Halfcar_model_EV_simulink/Wheel_rear/Tire Force_modi/If Action Subsystem ==
  Action Port : ActionPort  ActionType=then
  Constant : Constant  Value=0  OutDataType=fixdt(1, 16)  OutScaling=2^0  SampleTime=T
  Out1 : Outport  OutDataType=fixdt(1, 16)  OutScaling=2^0  InitialOutput=0
  wires:
  Constant/1 -> Out1/1

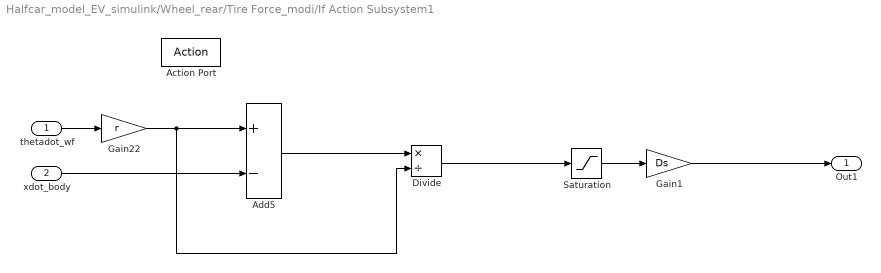
== system Halfcar_model_EV_simulink/Wheel_rear/Tire Force_modi/If Action Subsystem1 ==
  thetadot_wf : Inport
  xdot_body : Inport  Port=2
  Action Port : ActionPort  ActionType=elseif
  Add5 : Sum  Inputs=+-  OutDataType=fixdt(1, 16)  OutScaling=2^-10  SampleTime=T
  Divide : Product  Inputs=*/  OutDataType=fixdt(1, 16)  OutScaling=2^-10  SampleTime=T
  Gain1 : Gain  Gain=Ds  ParameterDataType=fixdt(1, 16)  ParameterScaling=2^0  OutDataType=fixdt(1, 16)  OutScaling=2^0  SampleTime=T
  Gain22 : Gain  Gain=r  ParameterDataType=fixdt(1, 16)  ParameterScaling=2^0  OutDataType=fixdt(1, 16)  OutScaling=2^0  SampleTime=T
  Saturation : Saturate  UpperLimit=saturation_slipratio  LowerLimit=-saturation_slipratio  SampleTime=T  OutDataType=fixdt(1, 16)  OutScaling=2^0
  Out1 : Outport  OutDataType=fixdt(1, 16)  OutScaling=2^0  InitialOutput=0
  wires:
  thetadot_wf/1 -> Gain22/1
  xdot_body/1 -> Add5/2
  Add5/1 -> Divide/1
  Divide/1 -> Saturation/1
  Gain22/1 -> Add5/1, Divide/2
  Saturation/1 -> Gain1/1
  Gain1/1 -> Out1/1

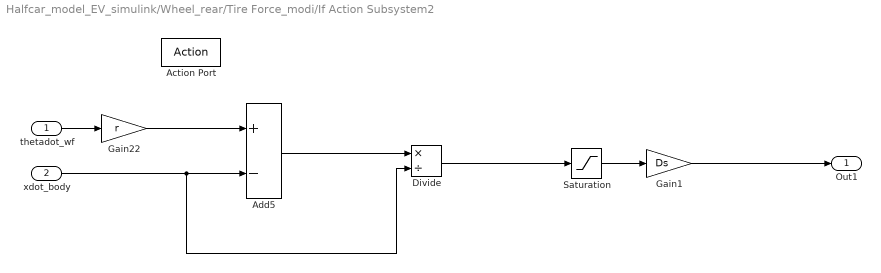
== system Halfcar_model_EV_simulink/Wheel_rear/Tire Force_modi/If Action Subsystem2 ==
  thetadot_wf : Inport
  xdot_body : Inport  Port=2
  Action Port : ActionPort  ActionType=else
  Add5 : Sum  Inputs=+-  OutDataType=fixdt(1, 16)  OutScaling=2^-10  SampleTime=T
  Divide : Product  Inputs=*/  OutDataType=fixdt(1, 16)  OutScaling=2^-10  SampleTime=T
  Gain1 : Gain  Gain=Ds  ParameterDataType=fixdt(1, 16)  ParameterScaling=2^0  OutDataType=fixdt(1, 16)  OutScaling=2^0  SampleTime=T
  Gain22 : Gain  Gain=r  ParameterDataType=fixdt(1, 16)  ParameterScaling=2^0  OutDataType=fixdt(1, 16)  OutScaling=2^0  SampleTime=T
  Saturation : Saturate  UpperLimit=saturation_slipratio  LowerLimit=-saturation_slipratio  SampleTime=T  OutDataType=fixdt(1, 16)  OutScaling=2^0
  Out1 : Outport  OutDataType=fixdt(1, 16)  OutScaling=2^0  InitialOutput=0
  wires:
  Gain1/1 -> Out1/1
  Saturation/1 -> Gain1/1
  Gain22/1 -> Add5/1
  Divide/1 -> Saturation/1
  Add5/1 -> Divide/1
  xdot_body/1 -> Add5/2, Divide/2
  thetadot_wf/1 -> Gain22/1
